simulink model "EMD_model_2"  (R2019a)
settings: Solver=ode45  StartTime=0  StopTime=setStopTime  FixedStep=0.0005  RelTol=1e-3  EnableMultiTasking=on
model workspace (MAT data in the model file):
  Body = timeseries
  Body.Name = 'unnamed'
  Body.DataInfo = tsdata.datametadata
  Body.DataInfo.Interpolation = tsdata.interpolation
  Body.DataInfo.Interpolation.Fhandle : function handle (value not decoded)
  Body.DataInfo.Interpolation.Name = 'linear'
  Body.TimeInfo = tsdata.timemetadata
  Body.TimeInfo.Length = 1
  Body.TimeInfo.DuplicateTimes = 0
  Body.TimeInfo.Time_ = 0
  Body.TimeInfo.Initialized = 1
  Body.QualityInfo = tsdata.qualmetadata
  Body.Data_ = 0
  Head = timeseries
  Head.Name = 'unnamed'
  Head.DataInfo = tsdata.datametadata
  Head.DataInfo.Interpolation = tsdata.interpolation
  Head.DataInfo.Interpolation.Fhandle : function handle (value not decoded)
  Head.DataInfo.Interpolation.Name = 'linear'
  Head.TimeInfo = tsdata.timemetadata
  Head.TimeInfo.Length = 1
  Head.TimeInfo.DuplicateTimes = 0
  Head.TimeInfo.Time_ = 0
  Head.TimeInfo.Initialized = 1
  Head.QualityInfo = tsdata.qualmetadata
  Head.Data_ = 0
  Stimulus = timeseries
  Stimulus.Name = 'unnamed'
  Stimulus.DataInfo = tsdata.datametadata
  Stimulus.DataInfo.Interpolation = tsdata.interpolation
  Stimulus.DataInfo.Interpolation.Fhandle : function handle (value not decoded)
  Stimulus.DataInfo.Interpolation.Name = 'linear'
  Stimulus.TimeInfo = tsdata.timemetadata
  Stimulus.TimeInfo.Length = 101
  Stimulus.TimeInfo.DuplicateTimes = 0
  Stimulus.TimeInfo.Time_ = [10; 10.1; 10.2; 10.3; 10.4; 10.5; 10.6; 10.7; 10.8; 10.9; 11; 11.1; 11.2; 11.3; 11.4; 11.5; 11.6; 11.7; 11.8; 11.9; 12; 12.1; 12.2; 12.3; 12.4; 12.5; 12.6; 12.7; 12.8; 12.9; 13; 13.1; 13.2; 13.3; 13.4; 13.5; 13.6; 13.7; 13.8; 13.9; 14; 14.1; 14.2; 14.3; 14.4; 14.5; 14.6; 14.7; 14.8; 14.9; 15; 15.1; 15.2; 15.3; 15.4; 15.5; 15.6; 15.7; 15.8; 15.9; 16; 16.1; 16.2; 16.3; 16.4; 16.5; 16.6; 16.7; 16.8; 16.9; 17; 17.1; 17.2; 17.3; 17.4; 17.5; 17.6; 17.7; 17.8; 17.9; 18; 18.1; 18.2; 18.3; 18.4; 18.5; 18.6; 18.7; 18.8; 18.9; 19; 19.1; 19.2; 19.3; 19.4; 19.5; 19.6; 19.7; 19.8; 19.9; 20]
  Stimulus.TimeInfo.Initialized = 1
  Stimulus.QualityInfo = tsdata.qualmetadata
  Stimulus.Data_ = [-3.67394039744e-15; 0.94185779294; 1.87999850346; 2.81071971879; 3.73034830747; 4.63525491562; 5.52186829027; 6.38668937348; 7.22630511153; 8.03740192468; 8.81677878439; 9.56135984623; 10.2682065889; 10.9345294113; 11.5576986416; 12.1352549156; 12.6649188825; 13.1446002007; 13.572405787; 13.9466472883; 14.2658477444; 14.5287474169; 14.7343087609; 14.8817205197; 14.9704009264; 15; 14.9704009264; 14.8817205197; 14.7343087609; 14.5287474169; 14.2658477444; 13.9466472883; 13.572405787; 13.1446002007; 12.6649188825; 12.1352549156; 11.5576986416; 10.9345294113; 10.2682065889; 9.56135984623; 8.81677878439; 8.03740192468; 7.22630511153; 6.38668937348; 5.52186829027; 4.63525491562; 3.73034830747; 2.81071971879; 1.87999850346; 0.94185779294; 5.51091059616e-15; -0.94185779294; -1.87999850346; -2.81071971879; -3.73034830747; -4.63525491562; -5.52186829027; -6.38668937348; -7.22630511153; -8.03740192468; -8.81677878439; -9.56135984623; -10.2682065889; -10.9345294113; -11.5576986416; -12.1352549156; -12.6649188825; -13.1446002007; -13.572405787; -13.9466472883; -14.2658477444; -14.5287474169; -14.7343087609; -14.8817205197; -14.9704009264; -15; -14.9704009264; -14.8817205197; -14.7343087609; -14.5287474169; -14.2658477444; -13.9466472883; -13.572405787; -13.1446002007; -12.6649188825; -12.1352549156; -11.5576986416; -10.9345294113; -10.2682065889; -9.56135984623; -8.81677878439; -8.03740192468; -7.22630511153; -6.38668937348; -5.52186829027; -4.63525491562; -3.73034830747; -2.81071971879; -1.87999850346; -0.94185779294; -7.34788079488e-15]
  bodyAmp = 0
  bodyPhase = 0
  freq = 0.628318530718
  headAmp = 0
  headPhase = 0
  high_delay = 0
  imageData = [0.00228480667088 0.00685422825671 0.0114230745906 0.0159909622235 0.0205575077854 0.0251223280162 0.0296850397975 0.0342452601838 0.0388026064343 0.0433566960441 0.0479071467754 0.0524535766893 ... (8204 elements, 1x8204)]
  low_delay = 0.035
  outputTimeList = [10; 10.1; 10.2; 10.3; 10.4; 10.5; 10.6; 10.7; 10.8; 10.9; 11; 11.1; 11.2; 11.3; 11.4; 11.5; 11.6; 11.7; 11.8; 11.9; 12; 12.1; 12.2; 12.3; 12.4; 12.5; 12.6; 12.7; 12.8; 12.9; 13; 13.1; 13.2; 13.3; 13.4; 13.5; 13.6; 13.7; 13.8; 13.9; 14; 14.1; 14.2; 14.3; 14.4; 14.5; 14.6; 14.7; 14.8; 14.9; 15; 15.1; 15.2; 15.3; 15.4; 15.5; 15.6; 15.7; 15.8; 15.9; 16; 16.1; 16.2; 16.3; 16.4; 16.5; 16.6; 16.7; 16.8; 16.9; 17; 17.1; 17.2; 17.3; 17.4; 17.5; 17.6; 17.7; 17.8; 17.9; 18; 18.1; 18.2; 18.3; 18.4; 18.5; 18.6; 18.7; 18.8; 18.9; 19; 19.1; 19.2; 19.3; 19.4; 19.5; 19.6; 19.7; 19.8; 19.9; 20]
  photo_a = [1 280.74949398 32070.4687612 642041.021699]
  photo_b = [0 0 0 1204751481.42]
  setStartTime = 5.68986602902
  setStopTime = 20
  stimAmp = 15
  temporalFilt = 0.035
  timeConstant = 0.06
libraries: visionsources x1
(part 1 of 2)
settings Model: SimulationMode=accelerator  Creator=Shane  LastModifiedBy=BC
settings DataIOCC: SaveFormat=Array  OutputOption=SpecifiedOutputTimes  OutputTimes=outputTimeList
settings OptimizationCC: ExpressionDepthLimit=2147483647  EfficientMapNaN2IntZero=off  SimCompilerOptimization=on
settings DebuggingCC: UnderspecifiedInitializationDetection=Classic  MergeDetectMultiDrivingBlocksExec=none  FcnCallInpInsideContextMsg=warning  StateNameClashWarn=warning  SFUnexpectedBacktrackingDiag=warning  SFNoUnconditionalDefaultTransitionDiag=warning  SFExecutionAtInitializationDiag=none  ArithmeticOperatorsInVariantConditions=warning
settings HardwareCC: ProdBitPerPointer=32  ProdBitPerSizeT=32  ProdBitPerPtrDiffT=32  ProdLargestAtomicFloat=None  ProdIntDivRoundTo=Undefined  ProdEndianess=Unspecified  ProdWordSize=32  ProdHWDeviceType=32-bit Generic  TargetBitPerPointer=64  TargetBitPerSizeT=64  TargetBitPerPtrDiffT=64  TargetLongLongMode=on  TargetIntDivRoundTo=Zero  TargetEndianess=LittleEndian  TargetWordSize=64  TargetHWDeviceType=MATLAB Host  ProdEqTarget=off
settings ModelReferenceCC: PropagateSignalLabelsOutOfModel=off
settings SFSimCC: SimUseLocalCustomCode=off
settings RTWCC: SystemTargetFile=accel.tlc  TemplateMakefile=accel_default_tmf  RTWVerbose=off
settings CodeAppCC: MaxIdLength=128
settings STFCustomTargetCC: ConcurrentExecutionCompliant=on  MATLABClassNameForMDSCustomization=Simulink.SoftwareTarget.TargetSpecificTriggerConfigurationBase  SystemTargetFile=accel.tlc
settings ConfigComp: CovMetricSettings=dw  CovHtmlReporting=on  CovSaveCumulativeToWorkspaceVar=on  CovSaveSingleToWorkspaceVar=on  CovExternalEMLEnable=off

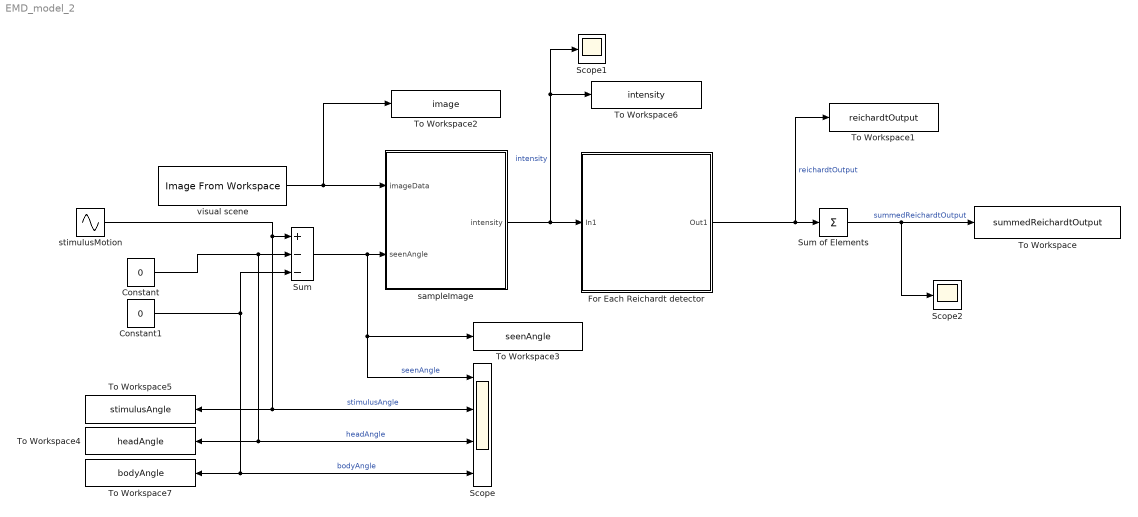
== system EMD_model_2 ==
  Constant : Constant  Value=0
  Constant1 : Constant  Value=0
  For Each Reichardt detector : Subsystem  TreatAsAtomicUnit=on
  Scope : Scope  NumInputPorts=4
  Scope1 : Scope
  Scope2 : Scope
  Sum : Sum  Inputs=+--
  Sum of Elements : Sum  Inputs=+
  To Workspace : ToWorkspace  VariableName=summedReichardtOutput  SaveFormat=Timeseries  SampleTime=-1
  To Workspace1 : ToWorkspace  VariableName=reichardtOutput  SaveFormat=Timeseries  SampleTime=-1
  To Workspace2 : ToWorkspace  VariableName=image  SaveFormat=Timeseries  SampleTime=-1
  To Workspace3 : ToWorkspace  VariableName=seenAngle  SaveFormat=Timeseries  SampleTime=-1
  To Workspace4 : ToWorkspace  VariableName=headAngle  SaveFormat=Timeseries  SampleTime=-1
  To Workspace5 : ToWorkspace  VariableName=stimulusAngle  SaveFormat=Timeseries  SampleTime=-1
  To Workspace6 : ToWorkspace  VariableName=intensity  SaveFormat=Timeseries  SampleTime=-1
  To Workspace7 : ToWorkspace  VariableName=bodyAngle  SaveFormat=Timeseries  SampleTime=-1
  sampleImage : MATLAB Function  TreatAsAtomicUnit=on
  stimulusMotion : Sin  Amplitude=stimAmp  Frequency=freq  SampleTime=0
  visual scene : visionsources/Image From Workspace  Tag=vipblks_nd  ImageValue=imageData  Ts=inf  imagePorts=One multidimensional signal  OutPortLabels=R|G|B  ImageDataType=double  Signed=on  WordLength=16  sdImageDataType=sfix(16)  FractionLengthMode=User-defined  FractionLength=15
      settings: SourceProductName=Computer Vision Toolbox  SourceProductBaseCode=VP
  wires:
  For Each Reichardt detector/1(Out1) -> To Workspace1/1, Sum of Elements/1  "reichardtOutput"
  Sum of Elements/1 -> Scope2/1, To Workspace/1  "summedReichardtOutput"
  sampleImage/1(intensity) -> Scope1/1, To Workspace6/1, For Each Reichardt detector/1(In1)  "intensity"
  visual scene/1 -> To Workspace2/1, sampleImage/1(imageData)
  stimulusMotion/1 -> To Workspace5/1, Scope/2, Sum/1  "stimulusAngle"
  Constant/1 -> To Workspace4/1, Scope/3, Sum/2  "headAngle"
  Sum/1 -> Scope/1, To Workspace3/1, sampleImage/2(seenAngle)  "seenAngle"
  Constant1/1 -> Sum/3, To Workspace7/1, Scope/4  "bodyAngle"
